simulink model "modelPID"  (R2018a)
settings: Solver=ode4  StartTime=0.0  StopTime=20  FixedStep=0.001  RelTol=1e-3
values from neighbouring files (symbols this model uses):
  a = zeros(1,6)    [StewartPlatform.m]
  kd = 1.22/kp    (= 0.392282958199)    [controller.m]
  ki = 2.28/kp    (= 0.733118971061)    [controller.m]
  kp = 3.11    [controller.m]
undefined symbols (not defined in the file or in its folder): b, c, d, ts
settings Model: Creator=Stuart Lunt  LastModifiedBy=Stuart Lunt

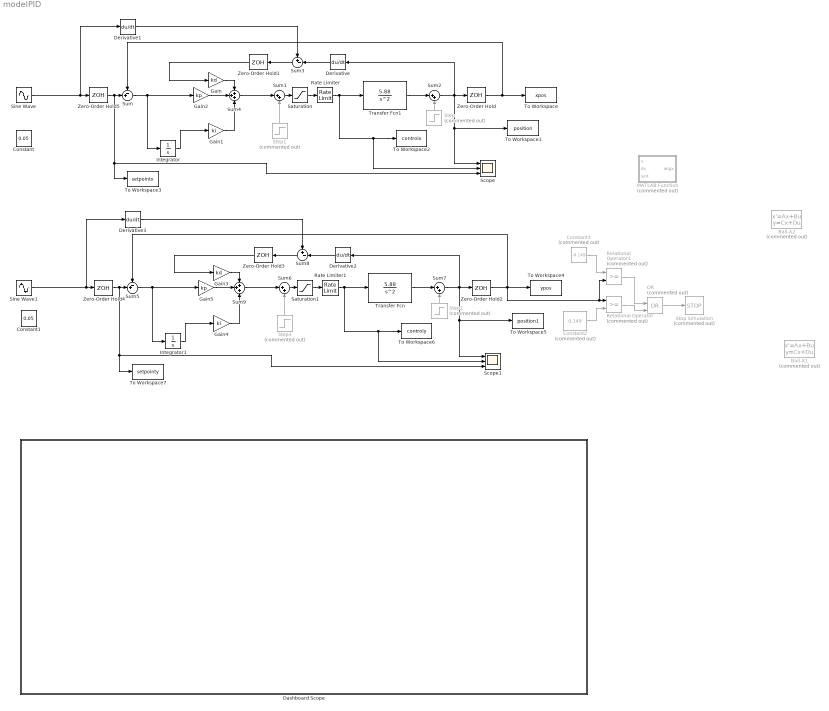
== system modelPID ==
  Ball-X1 : StateSpace  Commented=on  A=a  B=b  C=c  D=d  InitialCondition=0
  Ball-X2 : StateSpace  Commented=on  A=a  B=b  C=c  D=d  InitialCondition=0
  Constant : Constant  Value=0.05
  Constant1 : Constant  Value=0.05
  Constant2 : Constant  Commented=on  Value=0.149
  Constant3 : Constant  Commented=on  Value=-0.149
  Dashboard Scope : Subsystem  DialogController=hmiCreateDDGDialog  IsWebBlock=on  mask(MWDashboardBlock){webBlockId=eb3e894a-1342-41d6-8962-0bebce060ffb, webBlockType=sdiscope, ShowInitialText=on, HMISrcModelName=modelPID}
      mask prompts: webBlockId "WebBlock Id"; webBlockType "WebBlock Type"; HMISrcModelName "Source Model"
      mask help: SimulinkHMI:dialogs:HMIScopeDialogDesc
      mask Help: helpview([docroot '/mapfiles/simulink.map'], 'hmi_scope')
      mask Display:
      | if strcmp(get_param(bdroot(gcb),'BlockDiagramType'), 'library')
      |     image([(matlabroot) '/toolbox/simulink/hmi/icons/DashboardScope.png']);
      | end
  Derivative : Derivative  CoefficientInTFapproximation=0.005
  Derivative1 : Derivative
  Derivative2 : Derivative  CoefficientInTFapproximation=0.005
  Derivative3 : Derivative
  Gain : Gain  Gain=kd
  Gain1 : Gain  Gain=ki
  Gain2 : Gain  Gain=kp
  Gain3 : Gain  Gain=kd
  Gain4 : Gain  Gain=ki
  Gain5 : Gain  Gain=kp
  Integrator : Integrator
  Integrator1 : Integrator
  MATLAB Function : MATLAB Function  Commented=on  TreatAsAtomicUnit=on
  OR : Logic  Commented=on  Operator=OR  IconShape=distinctive  AllPortsSameDT=off  OutDataTypeStr=boolean
  Rate Limiter : RateLimiter  RisingSlewLimit=5  FallingSlewLimit=-5  SampleTimeMode=inherited
  Rate Limiter1 : RateLimiter  RisingSlewLimit=5  FallingSlewLimit=-5  SampleTimeMode=inherited
  Relational Operator : RelationalOperator  Commented=on  OutDataTypeStr=boolean  RndMeth=Simplest
  Relational Operator1 : RelationalOperator  Commented=on  OutDataTypeStr=boolean  RndMeth=Simplest
  Saturation : Saturate  UpperLimit=0.262  LowerLimit=-0.262
  Saturation1 : Saturate  UpperLimit=0.262  LowerLimit=-0.262
  Scope : Scope  NumInputPorts=3
  Scope1 : Scope  NumInputPorts=3
  Sine Wave : Sin  Amplitude=0.1  SampleTime=0
  Sine Wave1 : Sin  Amplitude=0.1  Phase=-pi/2  SampleTime=0
  Step : Step  Commented=on  Time=5  After=0.15  SampleTime=0
  Step1 : Step  Commented=on  Time=10  After=pi/60  SampleTime=0
  Step2 : Step  Commented=on  Time=5  After=0.15  SampleTime=0
  Step3 : Step  Commented=on  Time=10  After=pi/60  SampleTime=0
  Stop Simulation : Stop  Commented=on
  Sum : Sum  Inputs=-+|
  Sum{1..2,6..7} (4 alike) : Sum  Inputs=|++
  Sum3 : Sum  Inputs=+-|
  Sum4 : Sum  Inputs=+++
  Sum5 : Sum  Inputs=-+|
  Sum8 : Sum  Inputs=+-|
  Sum9 : Sum  Inputs=+++
  To Workspace : ToWorkspace  VariableName=xpos  SaveFormat=Structure With Time  SampleTime=-1
  To Workspace1 : ToWorkspace  VariableName=position  SaveFormat=Structure With Time  SampleTime=-1
  To Workspace2 : ToWorkspace  VariableName=controlx  SaveFormat=Structure With Time  SampleTime=-1
  To Workspace3 : ToWorkspace  VariableName=setpointx  SaveFormat=Structure With Time  SampleTime=-1
  To Workspace4 : ToWorkspace  VariableName=ypos  SaveFormat=Structure With Time  SampleTime=-1
  To Workspace5 : ToWorkspace  VariableName=position1  SaveFormat=Structure With Time  SampleTime=-1
  To Workspace6 : ToWorkspace  VariableName=controly  SaveFormat=Structure With Time  SampleTime=-1
  To Workspace7 : ToWorkspace  VariableName=setpointy  SaveFormat=Structure With Time  SampleTime=-1
  Transfer Fcn : TransferFcn  Numerator=[5.88]  Denominator=[1 0 0]
  Transfer Fcn1 : TransferFcn  Numerator=[5.88]  Denominator=[1 0 0]
  Zero-Order Hold{,1..5} (6 alike) : ZeroOrderHold  SampleTime=ts
  wires:
  Zero-Order Hold/1 -> To Workspace/1, Sum/1
  Transfer Fcn1/1 -> Sum2/1
  Sum2/1 -> Derivative/1, Zero-Order Hold/1, Scope/1, To Workspace1/1
  Step/1 -> Sum2/2
  Saturation/1 -> Rate Limiter/1
  Sine Wave/1 -> Derivative1/1, Zero-Order Hold5/1
  Sum/1 -> Integrator/1, Gain2/1
  Integrator/1 -> Gain1/1
  Rate Limiter/1 -> Transfer Fcn1/1, To Workspace2/1, Scope/2
  Sum1/1 -> Saturation/1
  Step1/1 -> Sum1/2
  Derivative/1 -> Sum3/2
  Derivative1/1 -> Sum3/1
  Sum3/1 -> Zero-Order Hold1/1
  Zero-Order Hold1/1 -> Gain/1
  Sum4/1 -> Sum1/1
  Gain/1 -> Sum4/1
  Gain1/1 -> Sum4/3
  Gain2/1 -> Sum4/2
  Transfer Fcn/1 -> Sum7/1
  Gain5/1 -> Sum9/2
  Gain3/1 -> Sum9/1
  Sum6/1 -> Saturation1/1
  Sum8/1 -> Zero-Order Hold3/1
  Sum5/1 -> Integrator1/1, Gain5/1
  Sum9/1 -> Sum6/1
  Derivative2/1 -> Sum8/2
  Sum7/1 -> Derivative2/1, Zero-Order Hold2/1, Scope1/1, To Workspace5/1
  Gain4/1 -> Sum9/3
  Saturation1/1 -> Rate Limiter1/1
  Rate Limiter1/1 -> Transfer Fcn/1, To Workspace6/1, Scope1/2
  Step2/1 -> Sum7/2
  Zero-Order Hold3/1 -> Gain3/1
  Zero-Order Hold2/1 -> Relational Operator1/2, Relational Operator/1, To Workspace4/1, Sum5/1
  Sine Wave1/1 -> Derivative3/1, Zero-Order Hold4/1
  Step3/1 -> Sum6/2
  Integrator1/1 -> Gain4/1
  Derivative3/1 -> Sum8/1
  Constant2/1 -> Relational Operator/2
  OR/1 -> Stop Simulation/1
  Constant3/1 -> Relational Operator1/1
  Relational Operator/1 -> OR/2
  Relational Operator1/1 -> OR/1
  Zero-Order Hold4/1 -> To Workspace7/1, Scope1/3, Sum5/2
  Zero-Order Hold5/1 -> To Workspace3/1, Scope/3, Sum/2

== system modelPID/Dashboard Scope ==

== matlab function modelPID/MATLAB Function ==
  data: x input; angx output; dx input; xint input
function angx = fcn(x, dx, xint)
kp=118.28;
ki=82.7;%/kp; %3.79
kd=41.6;%/kp;%2.26

% angx=kp*(x+kd*dx+ki*xint);
angx=kp*x+kd*dx+ki*xint;
